simulink model "chatter_SDOF"  (R2025b)
settings: Solver=FixedStepAuto  StartTime=0.0  StopTime=2.0  FixedStep=1/8000  RelTol=1e-3
undefined symbols (not defined in the file): c, h0, k, m, tau
libraries: simulink x2
settings Model: Creator=alinb  LastModifiedBy=alinb
settings DataIOCC: SaveOutput=off

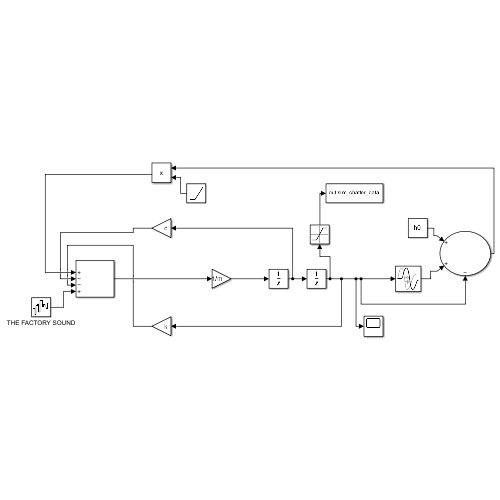
[thumbnail: Simulink's stored preview of the top-level diagram]
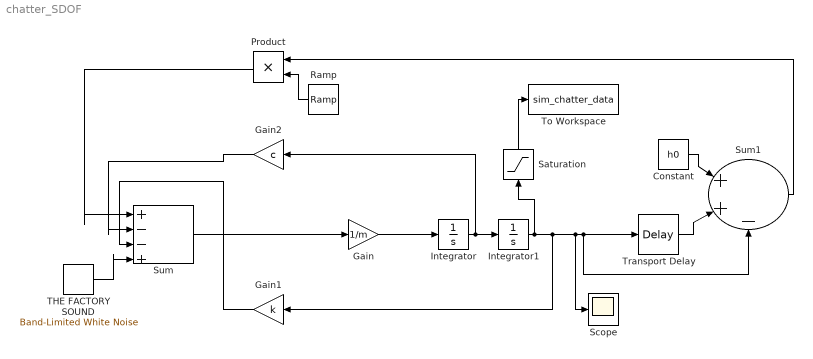
== system chatter_SDOF ==
  Constant : Constant  Value=h0
  Gain : Gain  Gain=1/m
  Gain1 : Gain  Gain=k
  Gain2 : Gain  Gain=c
  Integrator : Integrator
  Integrator1 : Integrator
  Product : Product
  Ramp : simulink/Sources/Ramp  slope=5e7  start=0  InitialOutput=0
  Saturation : Saturate  UpperLimit=0.005  LowerLimit=-0.005
  Scope : Scope
      settings: ActiveDisplayYMinimum=-0.00011485342442384078  ActiveDisplayYMaximum=0.000144500860294926
  Sum : Sum  Inputs=|+--+
  Sum1 : Sum  Inputs=|++-
  "THE FACTORY SOUND " : simulink/Sources/Band-Limited White Noise  Cov=1e-9  Ts=1/8000  seed=[23341]
  To Workspace : ToWorkspace  VariableName=sim_chatter_data  SampleTime=-1
  Transport Delay : TransportDelay  DelayTime=tau
  wires:
  Sum/1 -> Gain/1
  Gain/1 -> Integrator/1
  Integrator/1 -> Integrator1/1, Gain2/1
  Integrator1/1 -> Saturation/1, Scope/1, Sum1/3, Transport Delay/1, Gain1/1
  Gain2/1 -> Sum/2
  Gain1/1 -> Sum/3
  Transport Delay/1 -> Sum1/2
  Constant/1 -> Sum1/1
  Sum1/1 -> Product/1
  Product/1 -> Sum/1
  "THE FACTORY SOUND "/1 -> Sum/4
  Ramp/1 -> Product/2
  Saturation/1 -> To Workspace/1
